simulink model "programa_led"  (R2020b)
settings: Solver=VariableStepAuto  StartTime=0.0  StopTime=inf  RelTol=1e-3
undefined symbols (not defined in the file): serial
libraries: instrumentlib x2
settings Model: Creator=ashle  LastModifiedBy=cecir
settings SFSimCC: CustomCodeUndefinedFunction=UseInterfaceOnly

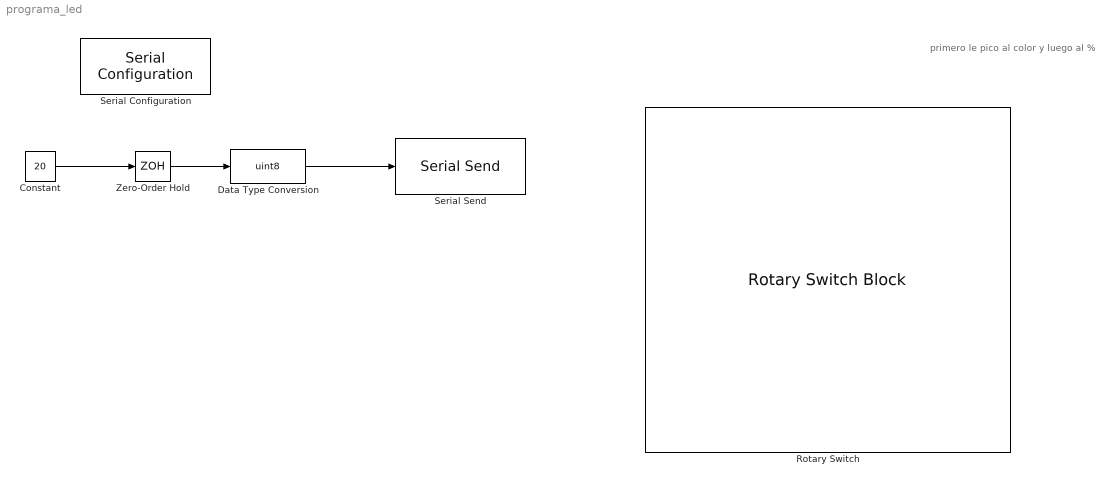
== system programa_led ==
  note: primero le pico al color y luego al %
  "Constant " : Constant  Value=20
  Data Type Conversion : DataTypeConversion  OutDataTypeStr=uint8
  Rotary Switch : RotarySwitchBlock
      settings: Values={{'0 %', '10 %', '20 %', '30 %', '40 %', '50 %', '60 %', '70 %', '80 %', '90 %', '100 %', 'R', 'A', 'V'}, [0 10 20 30 40 50 60 70 80 90 100 82 65 86]}
  "Serial Configuration " : instrumentlib/Serial Configuration  Priority=-200000  ComPortMenu=<Please select a port...>  ComPort=COM3  ObjConstructor=serial('COM3');  BaudRate=9600  DataBits=8  Parity=none  StopBits=1  FlowControl=none  Timeout=10  ByteOrder=LittleEndian
  "Serial Send " : instrumentlib/Serial Send  ComPortMenu=<Please select a port...>  ComPort=COM3  ObjConstructor=serial('COM3');  Terminator=<none>  EnableBlockingMode=on
  "Zero-Order Hold " : ZeroOrderHold  SampleTime=0.5
  wires:
  "Constant "/1 -> "Zero-Order Hold "/1
  "Zero-Order Hold "/1 -> Data Type Conversion/1
  Data Type Conversion/1 -> "Serial Send "/1
